simulink model "modeloFuzzy"  (Simulink 9.1)
settings: Solver=ode3  StartTime=0.0  StopTime=1  FixedStep=step  RelTol=1e-3  EnableMultiTasking=on
values from neighbouring files (symbols this model uses):
  D = 20    [ControleFuzzy.m]    (also in SistFuzzy.mat)
  delta = 3    [ControleFuzzy.m]
  gde = 20    [ControleFuzzy.m]    (also in SistFuzzy.mat)
  ge = 50    [ControleFuzzy.m]    (also in SistFuzzy.mat)
  gu = 100    [ControleFuzzy.m]    (also in SistFuzzy.mat)
  vari = 0.00001    (= 1e-05)    [ControleFuzzy.m]
libraries: simulink x3, fuzblock x1
settings Model: Creator=Zariff  LastModifiedBy=josen
settings DataIOCC: LimitDataPoints=on  SignalLoggingSaveFormat=ModelDataLogs
settings OptimizationCC: ExpressionDepthLimit=2147483647
settings DebuggingCC: SolverPrmCheckMsg=warning  FcnCallInpInsideContextMsg=warning  StateNameClashWarn=warning
settings GRTTargetCC: GeneratePreprocessorConditionals=Disable all

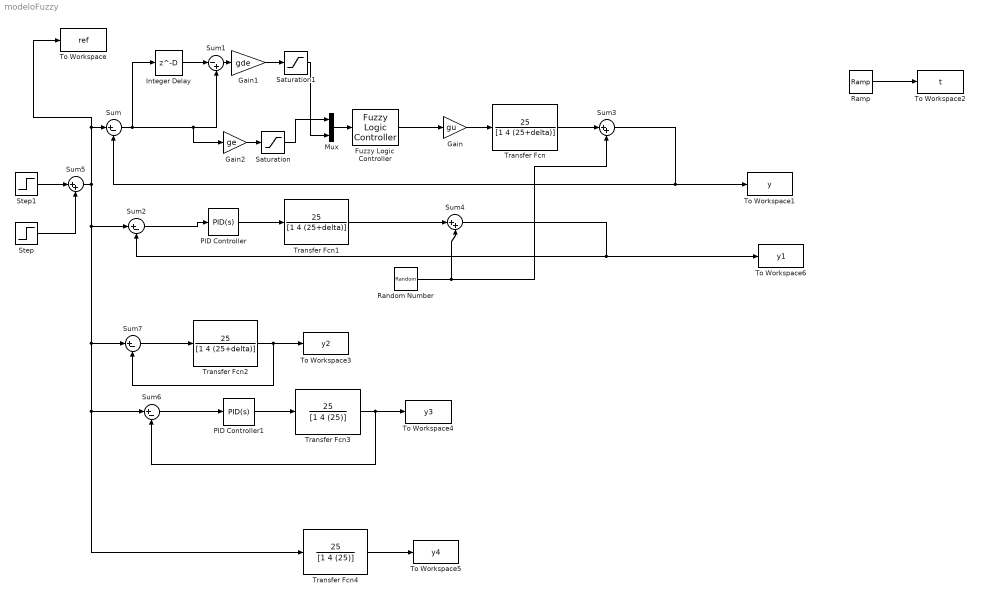
== system modeloFuzzy ==
  Fuzzy Logic  Controller : fuzblock/Fuzzy Logic  Controller  FIS=SistFuzzy  OutputSampleNumber=101  DataType=double  FuzzifiedInputs=off  RuleFiringStrengths=off  RuleOutputs=off  AggregatedOutputs=off  SimulateUsing=Interpreted execution  OutOfRangeInputValueMessage=warning  NoRuleFiredMessage=warning  EmptyOutputFuzzySetMessage=warning
  Gain : Gain  Gain=gu  OutDataTypeStr=Inherit: Same as input
  Gain1 : Gain  Gain=gde
  Gain2 : Gain  Gain=ge
  Integer Delay : Delay  DelayLength=D  SampleTime=0.0002
  Mux : Mux  Inputs=2
  PID Controller : simulink/Continuous/PID Controller  Controller=PID  TimeDomain=Continuous-time  SampleTime=-1  IntegratorMethod=Forward Euler  FilterMethod=Forward Euler  Form=Parallel  UseFilter=on  ControllerParametersSource=internal  P=4  I=25  D=1  N=100  InitialConditionSource=internal  InitialConditionForIntegrator=0  InitialConditionForFilter=0  ExternalReset=none  LimitOutput=off  UpperSaturationLimit=inf  LowerSaturationLimit=-inf  LinearizeAsGain=off  AntiWindupMode=none  Kb=1  TrackingMode=off  Kt=1  PParamMin=[]  PParamMax=[]  IParamMin=[]  IParamMax=[]  DParamMin=[]  DParamMax=[]  NParamMin=[]  NParamMax=[]  KbParamMin=[]  KbParamMax=[]  KtParamMin=[]  KtParamMax=[]  POutMin=[]  POutMax=[]  IOutMin=[]  IOutMax=[]  DOutMin=[]  DOutMax=[]  NOutMin=[]  NOutMax=[]  KbOutMin=[]  KbOutMax=[]  KtOutMin=[]  KtOutMax=[]  IntegratorOutMin=[]  IntegratorOutMax=[]  FilterOutMin=[]  FilterOutMax=[]  SumOutMin=[]  SumOutMax=[]  SumI1OutMin=[]  SumI1OutMax=[]  SumI2OutMin=[]  SumI2OutMax=[]  SumI3OutMin=[]  SumI3OutMax=[]  SumDOutMin=[]  SumDOutMax=[]  SaturationOutMin=[]  SaturationOutMax=[]  IntegratorContinuousStateAttributes=''  IntegratorStateMustResolveToSignalObject=off  IntegratorRTWStateStorageClass=Auto  FilterContinuousStateAttributes=''  FilterStateMustResolveToSignalObject=off  FilterRTWStateStorageClass=Auto  DifferentiatorICPrevScaledInput=0  DifferentiatorOutMin=[]  DifferentiatorOutMax=[]  FilterDiffOutCoefMin=[]  FilterDiffOutCoefMax=[]  SumDenOutMin=[]  SumDenOutMax=[]  SumNumOutMin=[]  SumNumOutMax=[]  ReciprocalOutMin=[]  ReciprocalOutMax=[]  DivideOutMin=[]  DivideOutMax=[]  TunerSelectOption=Transfer Function Based (PID Tuner App)
  PID Controller1 : simulink/Continuous/PID Controller  Controller=PID  TimeDomain=Continuous-time  SampleTime=-1  IntegratorMethod=Forward Euler  FilterMethod=Forward Euler  Form=Parallel  UseFilter=on  ControllerParametersSource=internal  P=4  I=25  D=1  N=100  InitialConditionSource=internal  InitialConditionForIntegrator=0  InitialConditionForFilter=0  ExternalReset=none  LimitOutput=off  UpperSaturationLimit=inf  LowerSaturationLimit=-inf  LinearizeAsGain=off  AntiWindupMode=none  Kb=1  TrackingMode=off  Kt=1  PParamMin=[]  PParamMax=[]  IParamMin=[]  IParamMax=[]  DParamMin=[]  DParamMax=[]  NParamMin=[]  NParamMax=[]  KbParamMin=[]  KbParamMax=[]  KtParamMin=[]  KtParamMax=[]  POutMin=[]  POutMax=[]  IOutMin=[]  IOutMax=[]  DOutMin=[]  DOutMax=[]  NOutMin=[]  NOutMax=[]  KbOutMin=[]  KbOutMax=[]  KtOutMin=[]  KtOutMax=[]  IntegratorOutMin=[]  IntegratorOutMax=[]  FilterOutMin=[]  FilterOutMax=[]  SumOutMin=[]  SumOutMax=[]  SumI1OutMin=[]  SumI1OutMax=[]  SumI2OutMin=[]  SumI2OutMax=[]  SumI3OutMin=[]  SumI3OutMax=[]  SumDOutMin=[]  SumDOutMax=[]  SaturationOutMin=[]  SaturationOutMax=[]  IntegratorContinuousStateAttributes=''  IntegratorStateMustResolveToSignalObject=off  IntegratorRTWStateStorageClass=Auto  FilterContinuousStateAttributes=''  FilterStateMustResolveToSignalObject=off  FilterRTWStateStorageClass=Auto  DifferentiatorICPrevScaledInput=0  DifferentiatorOutMin=[]  DifferentiatorOutMax=[]  FilterDiffOutCoefMin=[]  FilterDiffOutCoefMax=[]  SumDenOutMin=[]  SumDenOutMax=[]  SumNumOutMin=[]  SumNumOutMax=[]  ReciprocalOutMin=[]  ReciprocalOutMax=[]  DivideOutMin=[]  DivideOutMax=[]  TunerSelectOption=Transfer Function Based (PID Tuner App)
  Ramp : simulink/Sources/Ramp  slope=1  start=0  InitialOutput=0
  Random Number : RandomNumber  Variance=vari  SampleTime=0.0002
  Saturation : Saturate  UpperLimit=1  LowerLimit=-1
  Saturation1 : Saturate  UpperLimit=0.99  LowerLimit=-0.99
  Step : Step  Time=3.5  SampleTime=0
  Step1 : Step  Time=0  SampleTime=0
  Sum{,2,6..7} (4 alike) : Sum  Inputs=|+-
  Sum1 : Sum  Inputs=|-+
  Sum3 : Sum  Inputs=|++
  Sum4 : Sum  Inputs=|++
  Sum5 : Sum  Inputs=|++
  To Workspace : ToWorkspace  VariableName=ref  SampleTime=-1
  To Workspace1 : ToWorkspace  VariableName=y  SampleTime=-1
  To Workspace2 : ToWorkspace  VariableName=t  SampleTime=-1
  To Workspace3 : ToWorkspace  VariableName=y2  SampleTime=-1
  To Workspace4 : ToWorkspace  VariableName=y3  SampleTime=-1
  To Workspace5 : ToWorkspace  VariableName=y4  SampleTime=-1
  To Workspace6 : ToWorkspace  VariableName=y1  SampleTime=-1
  Transfer Fcn : TransferFcn  Numerator=[25]  Denominator=[1 4 (25+delta)]
  Transfer Fcn1 : TransferFcn  Numerator=[25]  Denominator=[1 4 (25+delta)]
  Transfer Fcn2 : TransferFcn  Numerator=[25]  Denominator=[1 4 (25+delta)]
  Transfer Fcn3 : TransferFcn  Numerator=[25]  Denominator=[1 4 (25)]
  Transfer Fcn4 : TransferFcn  Numerator=[25]  Denominator=[1 4 (25)]
  wires:
  Sum/1 -> Integer Delay/1, Sum1/2, Gain2/1
  Integer Delay/1 -> Sum1/1
  Sum1/1 -> Gain1/1
  Ramp/1 -> To Workspace2/1
  Sum2/1 -> PID Controller/1
  Mux/1 -> Fuzzy Logic  Controller/1
  PID Controller/1 -> Transfer Fcn1/1
  Saturation/1 -> Mux/1
  Saturation1/1 -> Mux/2
  Gain/1 -> Transfer Fcn/1
  Gain1/1 -> Saturation1/1
  Gain2/1 -> Saturation/1
  Transfer Fcn1/1 -> Sum4/1
  Sum4/1 -> To Workspace6/1, Sum2/2
  Random Number/1 -> Sum3/2, Sum4/2
  Transfer Fcn/1 -> Sum3/1
  Sum3/1 -> To Workspace1/1, Sum/2
  Step1/1 -> Sum5/1
  Step/1 -> Sum5/2
  Sum5/1 -> To Workspace/1, Sum/1, Sum2/1, Transfer Fcn4/1, Sum6/1, Sum7/1
  Transfer Fcn2/1 -> To Workspace3/1, Sum7/2
  Transfer Fcn3/1 -> To Workspace4/1, Sum6/2
  PID Controller1/1 -> Transfer Fcn3/1
  Sum6/1 -> PID Controller1/1
  Sum7/1 -> Transfer Fcn2/1
  Transfer Fcn4/1 -> To Workspace5/1
  Fuzzy Logic  Controller/1 -> Gain/1
